simulink model "plant2016_cybership_detectabl_switching"  (R2015b)
settings: Solver=VariableStepAuto  SolverMode=SingleTasking  StartTime=0.0  StopTime=200  FixedStep=.01  RelTol=1e-3  AbsTol=1e-6
StartFcn:
  | %plot_Contr_index('open')
libraries: simulink x9
(part 2 of 2)

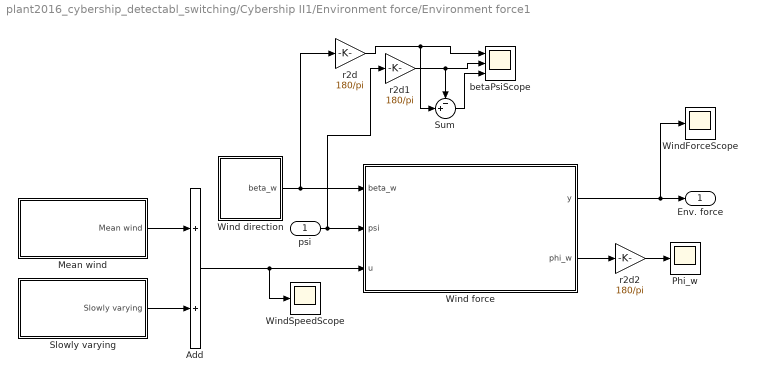
== system plant2016_cybership_detectabl_switching/Cybership II1/Environment force/Environment force1 ==
  psi : Inport
  Add : Sum  Inputs=2
  Mean wind : Subsystem  mask{windStrength=1, start=20}
      mask prompts: windStrength "Wind Strength"; start "Start Time"
  Phi_w : Scope
  Slowly varying : Subsystem  mask{start=25}
      mask prompts: start "Start Time"
  Sum : Sum  Inputs=-+|
  Wind direction : Subsystem
  Wind force : MATLAB Function  TreatAsAtomicUnit=on
  WindForceScope : Scope
  WindSpeedScope : Scope
  betaPsiScope : Scope  NumInputPorts=3
  r2d : Gain  Gain=180/pi
  r2d1 : Gain  Gain=180/pi
  r2d2 : Gain  Gain=180/pi
  Env. force : Outport
  wires:
  Add/1 -> WindSpeedScope/1, Wind force/3(u)
  Wind force/1(y) -> WindForceScope/1, Env. force/1
  psi/1 -> r2d1/1, Wind force/2(psi)
  Wind direction/1(beta_w) -> r2d/1, Wind force/1(beta_w)
  r2d/1 -> Sum/2, betaPsiScope/1
  Mean wind/1(Mean wind) -> Add/1
  Slowly varying/1(Slowly varying) -> Add/2
  r2d1/1 -> betaPsiScope/2, Sum/1
  Wind force/2(phi_w) -> r2d2/1
  r2d2/1 -> Phi_w/1
  Sum/1 -> betaPsiScope/3

== system plant2016_cybership_detectabl_switching/Cybership II1/Subsystem1/Subsystem ==
  A : Gain  Gain=[0 , 0 , 0 , 1 , 0 , 0 ; 0 , 0 , 0 , 0 , 1 , 0 ; 0 , 0 , 0 , 0 , 0 , 1 ; -omega_01^2 , 0 , 0 , -2*zeta_01*omega_01 , 0 , 0 ; 0 ,- omega_02^2 , 0 , 0 , -2*zeta_02*omega_02 , 0 ; 0 , 0 , -omega_03^2 , 0 , 0 , -2*zeta_03*omega_03]  Multiplication=Matrix(K*u) (u vector)
  Band-Limited White Noise1 : simulink/Sources/Band-Limited White Noise  Cov=[0.01;0.01;0.01]  Ts=0.1  seed=[23341]
  C : Gain  Gain=[zeros(3,3),eye(3)]  Multiplication=Matrix(K*u) (u vector)
  E : Gain  Gain=[zeros(3,3);eye(3)]  Multiplication=Matrix(K*u) (u vector)
  Integrator : Integrator  InitialCondition=[0;0;0;0;0;0]
  Product : Product
  Reference filter : Subsystem  mask(2nd order lop pass filter){omega_0=0.4, zeta=1}
      mask prompts: omega_0 "Critical frequency"; zeta "Damping ratio"
      mask help: The masked subsystem is a 2nd order linear siso low-pass filter with parameters set in the edit boxes
      mask Display: disp('2nd order LP')
  Scope : Scope
  Scope1 : Scope
  Step : Step  Time=start_time  SampleTime=0
  Sum : Sum  Inputs=|++
  1st order waves : Outport
  wires:
  Band-Limited White Noise1/1 -> E/1
  A/1 -> Integrator/1
  Integrator/1 -> Sum/2, C/1
  Sum/1 -> A/1
  E/1 -> Sum/1
  C/1 -> Scope1/1, Product/2
  Step/1 -> Reference filter/1(r(t))
  Product/1 -> 1st order waves/1
  Reference filter/1(r) -> Scope/1, Product/1

== system plant2016_cybership_detectabl_switching/Data-driven controller surge/ /look under the subsystem to see how it works ==
  note: Ficticious Reference
      | Signal of individual
      | Candidate Controller
      | R_fict (n)
  note: n - Candidate Controller Index
  Y (t) : Inport
  U (t) : Inport  Port=2
  Cost / Performance Index Generator : S-Function  FunctionName=cost_func_detectable  Parameters=w1_n, w1_d, w2_n, w2_d, C_p, C_i, C_d  SFunctionDeploymentMode=off  EnableBusSupport=off
  Demux2 : Demux  Tag=surge_demux_2  Outputs=2
  Ficticious Reference Signal Generator : S-Function  FunctionName=surge_fic_ref  Parameters=C_p, C_i, C_d  SFunctionDeploymentMode=off  EnableBusSupport=off
  Mux. : Mux  Inputs=2
  Mux.. : Mux  Inputs=2
  Mux2 : Mux  Tag=surge_mux_2  Inputs=2
  To Workspace : ToWorkspace  VariableName=surge_frs  SaveFormat=Timeseries  SampleTime=-1
  To Workspace1 : ToWorkspace  VariableName=surge_cost  SaveFormat=Timeseries  SampleTime=-1
  Out1 : Outport
  frs : Outport  Port=2
  wires:
  U (t)/1 -> Mux../1
  Mux./1 -> Cost / Performance Index Generator/1  "(u(t), y(t),r_fict(t))"
  Mux../1 -> Ficticious Reference Signal Generator/1, Mux./1  "U & Y"
  Y (t)/1 -> Mux../2
  Ficticious Reference Signal Generator/1 -> frs/1, To Workspace/1, Demux2/1
  Mux2/1 -> Mux./2  "R_Fict ( n x 1 )"
  Cost / Performance Index Generator/1 -> To Workspace1/1, Out1/1  "Performance Index of  each candidate controller (n x 1)"
  Demux2/1 -> Mux2/1
  Demux2/2 -> Mux2/2

== system plant2016_cybership_detectabl_switching/Data-driven controller surge/Adaptive  PID Controller/Approximate Derivative ==
  New State : Inport
  Trigger Signal : Inport  Port=2
  Y (t) : Inport  Port=3
  A : Gain  Gain=1/epsilon  SaturateOnIntegerOverflow=on  OutDataTypeStr=Inherit: Same as input  ParamDataTypeStr=Inherit: Same as input
  B : Gain  SaturateOnIntegerOverflow=on  OutDataTypeStr=Inherit: Same as input  ParamDataTypeStr=Inherit: Same as input
  C : Gain  Gain=-1/epsilon^2  SaturateOnIntegerOverflow=on  OutDataTypeStr=Inherit: Same as input  ParamDataTypeStr=Inherit: Same as input
  D : Gain  Gain=1/epsilon  SaturateOnIntegerOverflow=on  OutDataTypeStr=Inherit: Same as input  ParamDataTypeStr=Inherit: Same as input
  Integrator : Integrator  ExternalReset=either  InitialConditionSource=external
  Sum : Sum  Inputs=|+-
  Sum1 : Sum  Inputs=++|
  Out : Outport
  Derivative State : Outport  Port=2
  wires:
  Sum/1 -> Integrator/1
  Y (t)/1 -> D/1, B/1
  D/1 -> Sum1/1
  A/1 -> Sum/2
  Sum1/1 -> Out/1
  New State/1 -> Integrator/3
  Trigger Signal/1 -> Integrator/2
  C/1 -> Sum1/2
  Integrator/1 -> A/1, Derivative State/1, C/1
  B/1 -> Sum/1

== system plant2016_cybership_detectabl_switching/Data-driven controller sway/ /look under the subsystem to see how it works ==
  note: n - Candidate Controller Index
  note: Ficticious Reference
      | Signal of individual
      | Candidate Controller
      | R_fict (n)
  Y (t) : Inport
  U (t) : Inport  Port=2
  Cost / Performance Index Generator : S-Function  FunctionName=sway_cost_func  Parameters=w1_n, w1_d, w2_n, w2_d, C_p, C_i, C_d  SFunctionDeploymentMode=off  EnableBusSupport=off
  Demux2 : Demux  Tag=sway_demux_2  Outputs=1
  Ficticious Reference Signal Generator : S-Function  FunctionName=sway_fic_ref  Parameters=C_p, C_i, C_d  SFunctionDeploymentMode=off  EnableBusSupport=off
  Mux. : Mux  Inputs=2
  Mux.. : Mux  Inputs=2
  Mux2 : Mux  Tag=sway_mux_2  Inputs=1
  To Workspace : ToWorkspace  VariableName=sway_frs  SaveFormat=Timeseries  SampleTime=-1
  To Workspace1 : ToWorkspace  VariableName=sway_cost  SaveFormat=Timeseries  SampleTime=-1
  Out1 : Outport
  frs : Outport  Port=2
  wires:
  Cost / Performance Index Generator/1 -> Out1/1, To Workspace1/1  "Performance Index of  each candidate controller (n x 1)"
  Mux2/1 -> Mux./2  "R_Fict ( n x 1 )"
  Ficticious Reference Signal Generator/1 -> Demux2/1, To Workspace/1, frs/1
  Y (t)/1 -> Mux../2
  Mux../1 -> Mux./1, Ficticious Reference Signal Generator/1  "U & Y"
  Mux./1 -> Cost / Performance Index Generator/1  "(r_fict(t), u(t), y(t))"
  U (t)/1 -> Mux../1
  Demux2/1 -> Mux2/1

== system plant2016_cybership_detectabl_switching/Data-driven controller sway/Adaptive  PID Controller/Approximate Derivative ==
  New State : Inport
  Trigger Signal : Inport  Port=2
  Y (t) : Inport  Port=3
  Gain : Gain  Gain=1/epsilon^2  SaturateOnIntegerOverflow=on  OutDataTypeStr=Inherit: Same as input  ParamDataTypeStr=Inherit: Same as input
  Gain1 : Gain  Gain=1/epsilon  SaturateOnIntegerOverflow=on  OutDataTypeStr=Inherit: Same as input  ParamDataTypeStr=Inherit: Same as input
  Gain2 : Gain  Gain=1/epsilon  SaturateOnIntegerOverflow=on  OutDataTypeStr=Inherit: Same as input  ParamDataTypeStr=Inherit: Same as input
  Integrator : Integrator  ExternalReset=either  InitialConditionSource=external
  Sum : Sum  Inputs=+-  SaturateOnIntegerOverflow=on  InputSameDT=on  OutDataTypeStr=Inherit: Same as first input
  Sum1 : Sum  Inputs=+-  SaturateOnIntegerOverflow=on  InputSameDT=on  OutDataTypeStr=Inherit: Same as first input
  Out : Outport
  Derivative State : Outport  Port=2
  wires:
  Integrator/1 -> Gain/1, Gain2/1, Derivative State/1
  Gain/1 -> Sum1/2
  Trigger Signal/1 -> Integrator/2
  New State/1 -> Integrator/3
  Sum1/1 -> Out/1
  Gain2/1 -> Sum/2
  Gain1/1 -> Sum1/1
  Y (t)/1 -> Sum/1, Gain1/1
  Sum/1 -> Integrator/1

== system plant2016_cybership_detectabl_switching/Data-driven controller yaw/ /look under the subsystem to see how it works ==
  note: Ficticious Reference
      | Signal of individual
      | Candidate Controller
      | R_fict (n)
  note: n - Candidate Controller Index
  Y (t) : Inport
  U (t) : Inport  Port=2
  Cost / Performance Index Generator : S-Function  FunctionName=yaw_cost_func  Parameters=w1_n, w1_d, w2_n, w2_d, C_p, C_i, C_d  SFunctionDeploymentMode=off  EnableBusSupport=off
  Demux2 : Demux  Tag=yaw_demux_2  Outputs=1
  Ficticious Reference Signal Generator : S-Function  FunctionName=yaw_fic_ref  Parameters=C_p, C_i, C_d  SFunctionDeploymentMode=off  EnableBusSupport=off
  Mux. : Mux  Inputs=2
  Mux.. : Mux  Inputs=2
  Mux2 : Mux  Tag=yaw_mux_2  Inputs=1
  To Workspace : ToWorkspace  VariableName=yaw_frs  SaveFormat=Timeseries  SampleTime=-1
  To Workspace1 : ToWorkspace  VariableName=yaw_cost  SaveFormat=Timeseries  SampleTime=-1
  Out1 : Outport
  frs : Outport  Port=2
  wires:
  U (t)/1 -> Mux../1
  Mux./1 -> Cost / Performance Index Generator/1  "(r_fict(t), u(t), y(t))"
  Mux../1 -> Ficticious Reference Signal Generator/1, Mux./1  "U & Y"
  Y (t)/1 -> Mux../2
  Ficticious Reference Signal Generator/1 -> frs/1, To Workspace/1, Demux2/1
  Mux2/1 -> Mux./2  "R_Fict ( n x 1 )"
  Cost / Performance Index Generator/1 -> To Workspace1/1, Out1/1  "Performance Index of  each candidate controller (n x 1)"
  Demux2/1 -> Mux2/1

== system plant2016_cybership_detectabl_switching/Data-driven controller yaw/Adaptive  PID Controller/Approximate Derivative ==
  New State : Inport
  Trigger Signal : Inport  Port=2
  Y (t) : Inport  Port=3
  Gain : Gain  Gain=1/epsilon^2  SaturateOnIntegerOverflow=on  OutDataTypeStr=Inherit: Same as input  ParamDataTypeStr=Inherit: Same as input
  Gain1 : Gain  Gain=1/epsilon  SaturateOnIntegerOverflow=on  OutDataTypeStr=Inherit: Same as input  ParamDataTypeStr=Inherit: Same as input
  Gain2 : Gain  Gain=1/epsilon  SaturateOnIntegerOverflow=on  OutDataTypeStr=Inherit: Same as input  ParamDataTypeStr=Inherit: Same as input
  Integrator : Integrator  ExternalReset=either  InitialConditionSource=external
  Sum : Sum  Inputs=+-  SaturateOnIntegerOverflow=on  InputSameDT=on  OutDataTypeStr=Inherit: Same as first input
  Sum1 : Sum  Inputs=+-  SaturateOnIntegerOverflow=on  InputSameDT=on  OutDataTypeStr=Inherit: Same as first input
  Out : Outport
  Derivative State : Outport  Port=2
  wires:
  Sum/1 -> Integrator/1
  Y (t)/1 -> Gain1/1, Sum/1
  Gain1/1 -> Sum1/1
  Gain2/1 -> Sum/2
  Sum1/1 -> Out/1
  New State/1 -> Integrator/3
  Trigger Signal/1 -> Integrator/2
  Gain/1 -> Sum1/2
  Integrator/1 -> Derivative State/1, Gain2/1, Gain/1

== system plant2016_cybership_detectabl_switching/Cybership II/Environment force/Environment force1/Mean wind ==
  Constant4 : Constant  Value=windStrength
  Product : Product
  Reference filter : Subsystem
  Start1 : Step  Time=start  SampleTime=0
  Mean wind : Outport
  wires:
  Constant4/1 -> Product/2
  Start1/1 -> Product/1
  Reference filter/1(r) -> Mean wind/1  "mean_wind"
  Product/1 -> Reference filter/1(r(t))

== system plant2016_cybership_detectabl_switching/Cybership II/Environment force/Environment force1/Slowly varying ==
  1st order Markov2 : Subsystem
  Band-Limited White Noise1 : simulink/Sources/Band-Limited White Noise  Cov=1  Ts=0.1  seed=[23341]
  Product : Product
  Scope : Scope
  Start1 : Step  Time=100  SampleTime=0
  Slowly varying : Outport
  wires:
  Product/1 -> Scope/1, Slowly varying/1  "Slowly"
  Start1/1 -> Product/1
  1st order Markov2/1(Out1) -> Product/2
  Band-Limited White Noise1/1 -> 1st order Markov2/1(In1)

== system plant2016_cybership_detectabl_switching/Cybership II/Environment force/Environment force1/Wind direction ==
  1st order Markov1 : Subsystem
  Band-Limited White Noise1 : simulink/Sources/Band-Limited White Noise  Cov=10  Ts=0.1  seed=[23341]
  beta_w : Outport
  wires:
  1st order Markov1/1(Out1) -> beta_w/1
  Band-Limited White Noise1/1 -> 1st order Markov1/1(In1)

== system plant2016_cybership_detectabl_switching/Cybership II/Subsystem1/Subsystem/Reference filter ==
  r(t) : Inport
  2nd order LP1 : TransferFcn  Numerator=omega_0^2  Denominator=[1 2*zeta*omega_0 omega_0^2]
  r : Outport
  wires:
  r(t)/1 -> 2nd order LP1/1
  2nd order LP1/1 -> r/1

== system plant2016_cybership_detectabl_switching/Cybership II1/Environment force/Environment force1/Mean wind ==
  Constant4 : Constant  Value=windStrength
  Product : Product
  Reference filter : Subsystem
  Start1 : Step  Time=start  SampleTime=0
  Mean wind : Outport
  wires:
  Constant4/1 -> Product/2
  Start1/1 -> Product/1
  Reference filter/1(r) -> Mean wind/1  "mean_wind"
  Product/1 -> Reference filter/1(r(t))

== system plant2016_cybership_detectabl_switching/Cybership II1/Environment force/Environment force1/Slowly varying ==
  1st order Markov2 : Subsystem
  Band-Limited White Noise1 : simulink/Sources/Band-Limited White Noise  Cov=1  Ts=0.1  seed=[23341]
  Product : Product
  Reference filter : Subsystem
  Scope : Scope
  Start1 : Step  Time=100  SampleTime=0
  Slowly varying : Outport
  wires:
  Product/1 -> Reference filter/1(r(t))  "Slowly"
  Start1/1 -> Product/1
  1st order Markov2/1(Out1) -> Product/2
  Band-Limited White Noise1/1 -> 1st order Markov2/1(In1)
  Reference filter/1(r) -> Scope/1, Slowly varying/1

== system plant2016_cybership_detectabl_switching/Cybership II1/Environment force/Environment force1/Wind direction ==
  note: OBS: beta_w \in [0,360)
  1st order Markov2 : Subsystem
  Band-Limited White Noise1 : simulink/Sources/Band-Limited White Noise  Cov=10  Ts=0.1  seed=[23341]
  beta_w : Outport
  wires:
  1st order Markov2/1(Out1) -> beta_w/1
  Band-Limited White Noise1/1 -> 1st order Markov2/1(In1)

== system plant2016_cybership_detectabl_switching/Cybership II1/Subsystem1/Subsystem/Reference filter ==
  r(t) : Inport
  2nd order LP1 : TransferFcn  Numerator=omega_0^2  Denominator=[1 2*zeta*omega_0 omega_0^2]
  r : Outport
  wires:
  r(t)/1 -> 2nd order LP1/1
  2nd order LP1/1 -> r/1

== system plant2016_cybership_detectabl_switching/Cybership II/Environment force/Environment force1/Mean wind/Reference filter ==
  r(t) : Inport
  2nd order LP1 : TransferFcn  Numerator=0.4^2  Denominator=[1 2*1*0.4 0.4^2]
  r : Outport
  wires:
  r(t)/1 -> 2nd order LP1/1
  2nd order LP1/1 -> r/1

== system plant2016_cybership_detectabl_switching/Cybership II/Environment force/Environment force1/Slowly varying/1st order Markov2 ==
  In1 : Inport
  Gain : Gain  Gain=2
  Sum : Sum  Inputs=|+-
  Transfer Fcn : TransferFcn  Denominator=[50 1]
  Out1 : Outport
  wires:
  In1/1 -> Sum/1
  Sum/1 -> Transfer Fcn/1
  Transfer Fcn/1 -> Sum/2, Gain/1
  Gain/1 -> Out1/1

== system plant2016_cybership_detectabl_switching/Cybership II/Environment force/Environment force1/Wind direction/1st order Markov1 ==
  In1 : Inport
  2nd order LP1 : TransferFcn  Numerator=0.01^2  Denominator=[1 2*1*0.01 0.01^2]
  Constant : Constant  Value=pi*(2*rand()-1)
  Constant1 : Constant  Value=100
  Gain : Gain  Gain=2
  Sum : Sum  Inputs=|+-
  Sum1 : Sum  Inputs=++|
  Out1 : Outport
  wires:
  In1/1 -> Sum/1
  Sum/1 -> 2nd order LP1/1
  2nd order LP1/1 -> Gain/1
  Constant1/1 -> Sum1/1
  Gain/1 -> Sum1/2, Sum/2
  Sum1/1 -> Out1/1

== system plant2016_cybership_detectabl_switching/Cybership II1/Environment force/Environment force1/Mean wind/Reference filter ==
  r(t) : Inport
  2nd order LP1 : TransferFcn  Numerator=0.3^2  Denominator=[1 2*1*0.3 0.3^2]
  r : Outport
  wires:
  r(t)/1 -> 2nd order LP1/1
  2nd order LP1/1 -> r/1

== system plant2016_cybership_detectabl_switching/Cybership II1/Environment force/Environment force1/Slowly varying/1st order Markov2 ==
  In1 : Inport
  Gain : Gain  Gain=2
  Sum : Sum  Inputs=|+-
  Transfer Fcn : TransferFcn  Denominator=[50 1]
  Out1 : Outport
  wires:
  In1/1 -> Sum/1
  Sum/1 -> Transfer Fcn/1
  Transfer Fcn/1 -> Sum/2, Gain/1
  Gain/1 -> Out1/1

== system plant2016_cybership_detectabl_switching/Cybership II1/Environment force/Environment force1/Slowly varying/Reference filter ==
  r(t) : Inport
  2nd order LP1 : TransferFcn  Numerator=0.1^2  Denominator=[1 2*1*0.1 0.1^2]
  r : Outport
  wires:
  r(t)/1 -> 2nd order LP1/1
  2nd order LP1/1 -> r/1

== system plant2016_cybership_detectabl_switching/Cybership II1/Environment force/Environment force1/Wind direction/1st order Markov2 ==
  In1 : Inport
  2nd order LP1 : TransferFcn  Numerator=0.005^2  Denominator=[1 2*1*0.005 0.005^2]
  Constant : Constant  Commented=on  Value=2*pi*rand()
  Constant1 : Constant  Value=349.4*pi/180
  Gain : Gain  Gain=2
  Sum : Sum  Inputs=|+-
  Sum1 : Sum  Inputs=++|
  Out1 : Outport
  wires:
  In1/1 -> Sum/1
  Sum/1 -> 2nd order LP1/1
  2nd order LP1/1 -> Gain/1
  Constant1/1 -> Sum1/1
  Gain/1 -> Sum1/2, Sum/2
  Sum1/1 -> Out1/1

== matlab function plant2016_cybership_detectabl_switching/Data-driven controller surge/ /MATLAB Function1 ==
  data: frs input; y output; i input; y_sqr output
function [y,y_sqr] = fcn(frs,i)
%#codegen

y       = frs(i);
y_sqr   = frs.^2;

== matlab function plant2016_cybership_detectabl_switching/Data-driven controller surge/ /MATLAB Function ==
  data: cost input; y output; i input
function y = fcn(cost,i)
%#codegen

y = cost(i);

== matlab function plant2016_cybership_detectabl_switching/Data-driven controller surge/ /Selector ==
  data: u input; y output
function y = fcn(u)
%#codegen

y = u(4);

== matlab function plant2016_cybership_detectabl_switching/Cybership II/Path calculator ==
  data: tau input; nu input; nu_dot output
function nu_dot = fcn(tau,nu)
%% Cybership I
% % % m = 14.79;
% % % Iz = 1.76;
% % % xg = 0.0375;
% % % yg = 0;
% % % 
% % % Xudot   = -2;
% % % Yvdot   = -10;
% % % Yrdot   = 0;
% % % Nrdot   = -1;
% % % 
% % % Xu      = -0.4543;
% % % Yv      = -3.083;
% % % Yr      = -7.25;
% % % Nv      = 4.1117e-4;
% % % Nr      = -1.9;
% % % 
% % % M = [m-Xudot 0 0
% % %     0 m-Yvdot m*xg-Yrdot
% % %     0 m*xg - Yrdot Iz-Nrdot];
% % % 
% % % 
% % % D = [-Xu 0 0
% % %     0 -Yv -Yr    
% % %     0 -Nv -Nr];
% % % 
% % % nu_dot = -M\D*nu + M\tau;


%% Cybership II
% Data taken from: 
% @article{RN768,
%    author = {Hassani, Vahid and Pascoal, António M. and Aguiar, A. Pedro and Athans, Michael},
%    title = {A Multiple Model Adaptive Wave Filter for Dynamic Ship Positioning},
%    journal = {IFAC Proceedings Volumes},
%    volume = {43},
%    number = {20},
%    pages = {120-125},
%    ISSN = {1474-6670},
%    DOI = {http://dx.doi.org/10.3182/20100915-3-DE-3008.00026},
%    url = {http://www.sciencedirect.com/science/article/pii/S1474667016334486},
%    year = {2010},
%    type = {Journal Article}
% }


M = [   25.8,       0,          0;
        0,          33.8,       1.0115;
        0,          1.0115,     2.76];
    
D = [   2,          0,          0;
        0,          7,          0.1;
        0,          0.1,        0.5];

nu_dot = -M\D*nu + M\tau;

end

== matlab function plant2016_cybership_detectabl_switching/Data-driven controller surge/ /MATLAB Function2 ==
  data: u input; y output
function y  = fcn(u)
y=u^2;

== matlab function plant2016_cybership_detectabl_switching/Cybership II/eta_dot ==
  data: psi input; nu input; eta_dot output
function eta_dot = fcn(psi,nu)

R = [   cos(psi)    -sin(psi)   0
        sin(psi)     cos(psi)   0
        0            0          1];

eta_dot = R*nu;

end

== matlab function plant2016_cybership_detectabl_switching/Data-driven controller sway/ /MATLAB Function ==
  data: cost input; y output; i input
function y = fcn(cost,i)
%#codegen

y = cost(i);

== matlab function plant2016_cybership_detectabl_switching/Data-driven controller sway/ /MATLAB Function1 ==
  data: frs input; y output; i input; y_sqr output
function [y,y_sqr] = fcn(frs,i)
%#codegen

y       = frs(i);
y_sqr   = frs.^2;

== matlab function plant2016_cybership_detectabl_switching/Data-driven controller sway/ /MATLAB Function2 ==
  data: u input; y output
function y  = fcn(u)
y=u^2;

== matlab function plant2016_cybership_detectabl_switching/Data-driven controller sway/ /Selector ==
  data: u input; y output
function y = fcn(u)
%#codegen

y = u(5);

== matlab function plant2016_cybership_detectabl_switching/Data-driven controller yaw/ /MATLAB Function ==
  data: cost input; y output; i input
function y = fcn(cost,i)
%#codegen

y = cost(i);

== matlab function plant2016_cybership_detectabl_switching/Data-driven controller yaw/ /MATLAB Function1 ==
  data: frs input; y output; i input; y_sqr output
function [y,y_sqr] = fcn(frs,i)
%#codegen

y       = frs(i);
y_sqr   = frs.^2;

== matlab function plant2016_cybership_detectabl_switching/Data-driven controller yaw/ /MATLAB Function2 ==
  data: u input; y output
function y  = fcn(u)
y=u^2;

== matlab function plant2016_cybership_detectabl_switching/Data-driven controller yaw/ /Selector ==
  data: u input; y output
function y = fcn(u)
%#codegen

y = u(5);

== matlab function plant2016_cybership_detectabl_switching/Cybership II/Environment force/Environment force1/Wind force ==
  data: beta_w input; psi input; u input; y output
function y = fcn(beta_w,psi,u)
CX = 0.80;
CY = 1.00;
CN = 0.15;

phi_w = rad2pipi(-psi+beta_w);

R = [  -CX*cos(phi_w);
        CY*sin(phi_w);
        CN*sin(2*phi_w)];

y = u.*R;

== matlab function plant2016_cybership_detectabl_switching/Thrust allocation/NED2b ==
  data: tau input; tau_b output size=3; psi input
function tau_b = fcn(tau,psi)
R = [   cos(psi)    -sin(psi)   0
        sin(psi)     cos(psi)   0
        0            0          1];
tau_b = R'*tau;

== matlab function plant2016_cybership_detectabl_switching/Cybership II1/Environment force/Environment force1/Wind force ==
  data: beta_w input; psi input; u input; y output; phi_w output
function [y,phi_w] = fcn(beta_w,psi,u)
CX = 0.70;  % CX \in {0.50,0.90}
CY = 0.87;  % CY \in {0.70,0.95}
CN = 0.05;  % CN \in {0.05,0.20} - After reccomodations found on p.191 in Fossen

phi_w = rad2pipi(beta_w-psi);

R = [  -CX*cos(phi_w);
       -CY*sin(phi_w);
       -CN*sin(2*phi_w)];

y = u.*R;

== matlab function plant2016_cybership_detectabl_switching/Cybership II/MATLAB Function ==
  data: eta input; y output
function y = rad2pipi(eta)

angle = eta(3);
r = rem(angle+sign(angle)*pi,2*pi);
s = sign(sign(angle) + 2*(sign(abs(rem(angle+pi,2*pi)/(2*pi)))-1));

y = [   eta(1);
        eta(2);
        r - s*pi];

== matlab function plant2016_cybership_detectabl_switching/Cybership II1/Path calculator ==
  data: tau input; nu input; nu_dot output
function nu_dot = fcn(tau,nu)
%% Cybership I
% % % m = 14.79;
% % % Iz = 1.76;
% % % xg = 0.0375;
% % % yg = 0;
% % % 
% % % Xudot   = -2;
% % % Yvdot   = -10;
% % % Yrdot   = 0;
% % % Nrdot   = -1;
% % % 
% % % Xu      = -0.4543;
% % % Yv      = -3.083;
% % % Yr      = -7.25;
% % % Nv      = 4.1117e-4;
% % % Nr      = -1.9;
% % % 
% % % M = [m-Xudot 0 0
% % %     0 m-Yvdot m*xg-Yrdot
% % %     0 m*xg - Yrdot Iz-Nrdot];
% % % 
% % % 
% % % D = [-Xu 0 0
% % %     0 -Yv -Yr    
% % %     0 -Nv -Nr];
% % % 
% % % nu_dot = -M\D*nu + M\tau;


%% Cybership II
% Data taken from: 
% @article{RN768,
%    author = {Hassani, Vahid and Pascoal, António M. and Aguiar, A. Pedro and Athans, Michael},
%    title = {A Multiple Model Adaptive Wave Filter for Dynamic Ship Positioning},
%    journal = {IFAC Proceedings Volumes},
%    volume = {43},
%    number = {20},
%    pages = {120-125},
%    ISSN = {1474-6670},
%    DOI = {http://dx.doi.org/10.3182/20100915-3-DE-3008.00026},
%    url = {http://www.sciencedirect.com/science/article/pii/S1474667016334486},
%    year = {2010},
%    type = {Journal Article}
% }


M = [   25.8,       0,          0;
        0,          33.8,       1.0115;
        0,          1.0115,     2.76];
    
D = [   2,          0,          0;
        0,          7,          0.1;
        0,          0.1,        0.5];

nu_dot = -M\D*nu + M\tau;

end

== matlab function plant2016_cybership_detectabl_switching/Cybership II1/rad2pipi ==
  data: eta input; y output
function y = rad2pipi(eta)

angle = eta(3);
r = rem(angle+sign(angle)*pi,2*pi);
s = sign(sign(angle) + 2*(sign(abs(rem(angle+pi,2*pi)/(2*pi)))-1));

y = [   eta(1);
        eta(2);
        r - s*pi];

== matlab function plant2016_cybership_detectabl_switching/Cybership II1/eta_dot ==
  data: psi input; nu input; eta_dot output
function eta_dot = fcn(psi,nu)

R = [   cos(psi)    -sin(psi)   0
        sin(psi)     cos(psi)   0
        0            0          1];

eta_dot = R*nu;

end
